simulink model "uvms_sliding"  (Simulink 7.9)
settings: Solver=ode4  StartTime=0.0  StopTime=10.0  FixedStep=dt  RelTol=2*1e-3
values from neighbouring files (symbols this model uses):
  DH = struct('a',zeros(n,1),'d',zeros(n,1),'alpha',zeros(n,1))    [init.m]
  dt = 0.01    [run_simulation.m]
undefined symbols (not defined in the file or in its folder): commanded_zeta, ee_pose_init, Kinetics_Parameters, q_init, V_current, vehicle_euler_init, vehicle_position_init
(part 2 of 2)

== matlab function Controller/sliding mode 2/tau1 ==
  data: Kinetics_Parameters input Bus: kinetics_bus; tau output double; Kinematics input Bus: kin_bus; Measured_States input double; Commanded_States input double; dxi_com input double; dxi_mes input double; dzeta_0_com input double
function tau = slidingMode(Kinetics_Parameters, Kinematics,Measured_States,Commanded_States,dxi_com, dxi_mes, dzeta_0_com)
%#codegen
    Lambda = diag([ones(1,6)*25 , ones(1,6)*25]);
    zeta_mes = Measured_States.zeta;
    y = Lambda * (Commanded_States.xi - Measured_States.xi);
    zeta_0_tilde = dxi_com - dxi_mes;
    zeta_0_com = dxi_com;
    dy = Lambda * zeta_0_tilde;
    s = y + zeta_0_tilde;
    xi_mes = Measured_States.xi;
    
    % get the jacobian Ja
    R0b = Kinematics.Ti.R0b;
    Teuler = getTeuler( Measured_States.xi (4:6)  );
    Ja = [ R0b' , zeros(3,3), zeros(3,6);
           zeros(3,3), Teuler, zeros(3,6);
           zeros(6,3), zeros(6,3), eye(6)
         ];
    dJa = getdJa (Kinematics, zeta_mes, xi_mes, dxi_mes);
    
    N = getN (Kinematics,Kinetics_Parameters);
    M0 = 0.9*getM0 (Kinematics, Kinetics_Parameters, Ja);
    M = getM (Kinematics,Kinetics_Parameters);
    C0 = 1.1*getC0 (Kinematics,Kinetics_Parameters, zeta_mes , Ja, dJa);
    D0 = 1.1*getD0 (Kinematics, Kinetics_Parameters, zeta_mes , Ja);
    
       
    
    Kd=diag([ones(1,6)*60, ones(1,6)*50]);
    Ks=diag([ones(1,6)*390, ones(1,6)*300]);
    
    temp = (dy + dzeta_0_com);
    temp2 = (y + zeta_0_com);
    tau = M0* temp   +  M* dJa* s + C0* temp2 + D0* temp2 + N + Kd*Ja* s + Ks* sat(Ja*s, 0.05);  
    
    
end


function vec = sat (x,epsilon)
    vec=zeros(length(x),1);
    for i=1:length(x)
       if x(i) > epsilon
           vec(i)=1;
       elseif x(i) < -epsilon
           vec(i)=-1;
       else
           vec(i)=x(i)/epsilon;
       end
    end
end

% get the derivative of the jacobian matrix Ja
function dJa = getdJa(Kinematics, zeta, xi , dxi)
    Rb0 = Kinematics.Ti.R0b';
    omega0b = zeta(4:6);
    dRb0 = - Rb0 * skew (omega0b);
    dTb0 = getdTb0( xi, dxi);
    dJa = [ dRb0 , zeros(3,3), zeros(3,6);
           zeros(3,3), dTb0, zeros(3,6);
           zeros(6,3), zeros(6,3), zeros(6,6);
         ];
end

% get the derivative of the Transfromation matrix from euler rates to body
% rates
function dTb0 = getdTb0( xi, dxi)
    dTb0 = zeros(3,3);
    phi = xi(4);
    theta = xi(5);
    dphi = dxi(4);
    dtheta = dxi(5);
    
    dTb0 = [...
            0,           0,      - cos(theta)*dtheta;
            0,    -sin(phi)*dphi,   -sin(theta)*dtheta*sin(phi) + cos(theta)*cos(phi)*dphi;
            0,    -cos(phi)     ,   -sin(theta)*dtheta*cos(phi) - cos(theta)*sin(phi)*dphi
            ];
end

% Get the transformation matrix from euler rates to body rates
function T = getTeuler ( euler )
    phi=euler(1);
    theta=euler(2);
    psi=euler(3);
       
    cphi = cos(phi);
    sphi = sin(phi);
    cth  = cos(theta);
    sth  = sin(theta);
 
    T = [...
      1  0      -sth;
      0  cphi   cth*sphi;
      0  -sphi  cth*cphi ];
end



%% --------------------------------------------------------------
%  Functions to gather the vectors   
%%---------------------------------------------------------------

function M0 = getM0(Kinematics, Kinetics_Parameters, Ja)
    Mrb = getInertiaMatrix(Kinematics, Kinetics_Parameters);
    Ma = getMa(Kinematics, Kinetics_Parameters);
    M0 = (Mrb + Ma)*Ja;
end

function M = getM(Kinematics, Kinetics_Parameters)
    Mrb = getInertiaMatrix(Kinematics, Kinetics_Parameters);
    Ma = getMa(Kinematics, Kinetics_Parameters);
    M = (Mrb + Ma);
end


function C0 = getC0 (Kinematics,Kinetics_Parameters,zeta, Ja, dJa)
    C = getCrb(Kinematics,Kinetics_Parameters, zeta)  + getCa(Kinematics,Kinetics_Parameters,zeta);
    M = getM(Kinematics, Kinetics_Parameters);
    
    C0 = C*Ja + M*dJa;
end

function D0 = getD0 (Kinematics, Kinetics_Parameters,zeta, Ja)
    D =  getD(Kinematics, Kinetics_Parameters,zeta);
    D0 = D* Ja;
end


%% --------------------------------------------------------------
%  Inertia function   
%%---------------------------------------------------------------
function M = getInertiaMatrix(Kinematics, Kinetics_Parameters)
%#codegen
%   getInertiaMatrix Returns the sum of the Rigid body inertia and the added mass:
%   M_rb + M_a
%   
    n=6;
    i=1;
    M = zeros(12,12);
    Inertia = Kinetics_Parameters.Inertia;
    Jgb = [eye(6), zeros(6,6)];                                 % Jacobian from vehicle 
    Ji=Jgb;
    Hi = Kinetics_Parameters.Persistent.Hrg(:,:,i);
    Ii=Hi'*(Inertia(:,:,1))*Hi;                                 % Inertia of vehicle in CO
    M=M+(Ji')*Ii*Ji;
    for i=1:n
        Ji = Kinematics.Ji.Ji(:,:,i);                           % body jacobian
        Hi =Kinetics_Parameters.Persistent.Hrg(:,:,i+1);        % get Transformation matrix of link i
        Ii=Hi'*(Inertia(:,:,i+1) )*Hi;                          % Transform Inertia matrix from CG to CO
        M=M+(Ji')*Ii*Ji;                                        % Add link i's inertia to total inertia
    end
end







%% ------------------------------------------------------
% Persistent Forces   
%%-------------------------------------------------------
function N_p = getN(Kinematics,Kinetics_Parameters)
%#codegen
%   N_p - 12 x 1 vector of generalized forces
%   Persistent_Forces returns the generalized forces due to boyancy and 
%   gravity

    %% init
    n=6;
    N_p=zeros(12,1);
    Jgis = Kinematics.Ji.Ji;
    
    %%  vehicle
    F_bp = getFbp(Kinematics, Kinetics_Parameters,1);           % Get wrench from persistent forces in CO
    Jbb=([eye(6), zeros(6,6)]);                                 % Jacobian from b to b
    N_p = Jbb'*F_bp;                                            % Get contribution to total forces through Jbb
    
    %% robot links
    for i=1:n
        Jgi=Jgis(:,:,i);                                        % Jacobian from b to i
        F_ip = getFip(Kinematics,Kinetics_Parameters, i+1);     % Get wrench in CO
        N_p = N_p + (Jgi')*F_ip;                                % Map to generalized forces and add to total
    end
    N_p = - N_p;                                                % reverse the sign to comply with the sign convention
end
    
    
function F_ip = getFip(Kinematics,Kinetics_Parameters, i)
%#codegen
% function calculating wrench from persistent forces 
% i=b: vehicle
% i>=1: robot arms
    F_ip = zeros(6,1);
    mi = Kinetics_Parameters.Persistent.m(i);
    g = Kinetics_Parameters.Persistent.g;
    rho = Kinetics_Parameters.Persistent.rho;
    nabla = Kinetics_Parameters.Persistent.nabla(i);
    Ri0 = Kinematics.Ti.R0i(:,:,i-1)';
    Hrg = Kinetics_Parameters.Persistent.Hrg(:,:,i);  
    Hrb = Kinetics_Parameters.Persistent.Hrb(:,:,i);
    ez=[0;0;1];
    F_ip(:,:) = (Hrg')*[-mi*g*Ri0*ez ;0;0;0]  + (Hrb')*[rho*nabla*g*Ri0*ez ;0;0;0 ];
end


function F_bp = getFbp(Kinematics,Kinetics_Parameters, i)
%#codegen
% function calculating wrench from persistent forces 
% i=b: vehicle
% i>=1: robot arms
    F_bp = zeros(6,1);
    mi = Kinetics_Parameters.Persistent.m(i);
    g = Kinetics_Parameters.Persistent.g;
    Hrg = Kinetics_Parameters.Persistent.Hrg(:,:,i);  
    Hrb = Kinetics_Parameters.Persistent.Hrb(:,:,i);
    rho = Kinetics_Parameters.Persistent.rho;
    nabla = Kinetics_Parameters.Persistent.nabla(i);
    Ri0 = (Kinematics.Ti.R0b)';
    ez=[0;0;1];
    F_bp(:,:) = (Hrg')*[-mi*g*Ri0*ez ; 0;0;0]  + (Hrb')*[rho*nabla*g*Ri0*ez ; 0;0;0 ];
end

function [phi,theta,psi] = myR2euler(R)
%#codegen
    phi   = atan2(R(3,2),R(3,3));
    theta = -asin(R(3,1));
    psi   = atan2(R(2,1),R(1,1));
end



%% ------------------------------------------------------
% Coriolis Matrix   
%%-------------------------------------------------------
function C = getCrb(Kinematics,Kinetics_Parameters, zeta)
%#codegen
%-----------------------------------------------------------------------
%   This function calculates the coriolis according to From and Pettersen
%   (2013).
%-----------------------------------------------------------------------
    n=6;
    C=zeros(12,12);
    Inertia=Kinetics_Parameters.Inertia;
    Jis = Kinematics.Ji.Ji;
    
    % i = b
    Jgb = [eye(6), zeros(6,6)];
    i=1;
    Hi = Kinetics_Parameters.Persistent.Hrg(:,:,i);
    Ii=Hi'*Inertia(:,:,i);
    Wb = getWb(Ii,zeta);
    C = - (Jgb')*Wb*Hi*Jgb;     % time derivative of Jgb = 0  
    
    % i >=1
    for i=1:n
        Hi = Kinetics_Parameters.Persistent.Hrg(:,:,i+1);
        Ii=Hi'*Inertia(:,:,i+1);
        Wi=getWi(Ii,Jis(:,:,i), zeta);
        Jgi_dot=getJgi_dot(Kinematics, zeta,i);
        Jgi = Jis(:,:,i);
        
        C = C + (Jgi')*Ii*Hi*Jgi_dot - (Jgi')*Wi*Hi*Jgi;
    end
end



function Wb = getWb(I , zeta)
%#codegen
% Get the matrix Wi for i=b
% I: Inertia matrix for vehicle
% zeta: generalized velocity
    Wb = zeros(6,6);
    v = zeta(1:3);
    omega = zeta(4:6);
    mI = I(1:3,1:3); % Identity matrix times mass of link b
    Ib = I(4:6,4:6); % Moment of inertia
    mrgb = I(4:6,1:3); % mass times skew symmetric r_g^b
    dKv= mI*v - mrgb*omega;
    dKomega = Ib*omega + mrgb*v;
    
    Wb = [zeros(3,3), skew(dKv) ; skew(dKv), skew(dKomega)];
end

function Wi = getWi(I, Ji,zeta)
%#codegen
% Get matrix Wi for robot links
% I: inertia matrix for link i
% Ji: Jacobian for link i
% zeta: generalized coordinates
    Wi = zeros(6,6);
    V0i = Ji*zeta;
    v = V0i(1:3);
    omega = V0i(4:6);
    mI = I(1:3,1:3); % Identity matrix times mass of link b
    Ib = I(4:6,4:6); % Moment of inertia
    mrgb = I(4:6,1:3); % mass times skew symmetric r_g^b
    dKv= mI*v - mrgb*omega;
    dKomega = Ib*omega + mrgb*v;
    Wi = [zeros(3,3), skew(dKv) ; skew(dKv), skew(dKomega)];
end

function Jgi_dot=getJgi_dot(Kinematics, zeta,i)
%#codegen
% the functions below is related to Jgi_dot
    Jgi_dot = zeros(6,6+6);
    n=6;
    Jgi = Kinematics.Ji.Ji(:,:,i);
    omega = Jgi*zeta;
    Rbi = Kinematics.Ti.Rbi(:,:,i);
    pbi = Kinematics.Ti.pbi(:,i);
    omegaib = getOmegaib(Kinematics,zeta,i);
    dpbi =  getDpbi(Kinematics,zeta,i);
        
    dAdg_inv = [(Rbi')*skew(omegaib) , -(Rbi')*skew(omegaib)*skew(pbi) + (Rbi')*skew(dpbi); ...
                zeros(3,3) , (Rbi')*skew(omegaib) ];
    dJi = zeros(6,6);
    omega0b = zeta(4:6);
    
    % get d/dt(Ji)
    Xii=[0,0,0,0,0,1]';
    for k=2:n
       if k<=i
            dpbk = getDpbi(Kinematics, zeta ,k-1);
            Rbk= Kinematics.Ti.Rbi(:,:,k-1);
            omega0k = [zeros(3,3) , eye(3)]*Kinematics.Ji.Ji(:,:,k-1)*zeta;
            omegabk = omega0k - (Rbk')*omega0b;
            dJi(:,k) = [zeros(3,3), skew(dpbk)*Rbk*skew(omegabk) ...
                ; zeros(3,3) , (Rbk')*skew(omegabk)]*Xii;
       end
    end
    Ji=getji(Kinematics.Ti, i);
    Adg_inv = Kinematics.Ti.Adgbi_inv(:,:,i);
    Jgi_dot = [dAdg_inv, dAdg_inv*Ji + Adg_inv*dJi ];
end

function omegaib = getOmegaib(Kinematics,zeta,i)
%#codegen
% returns angular rage of vehcile wrt frame i noted in vehicle frame
    omegaib = zeros(3,1);
    Rbi = Kinematics.Ti.Rbi(:,:,i);
    Jgi = Kinematics.Ji.Ji(:,:,i);
    omega0b = zeta(4:6);
    omegaib = omega0b - Rbi*[zeros(3,3), eye(3)]*Jgi*zeta;
end

function dpbi = getDpbi( Kinematics, zeta,iter)
%#codegen
% returns time derivative of position vector of from frame b to frame i
    dpbi = zeros(3,1);
    H = [eye(3), zeros(3,3)];
    Rbi=Kinematics.Ti.Rbi(:,:,iter);
    Adgbi_inv = Kinematics.Ti.Adgbi_inv(:,:,iter);
    Ji = getji(Kinematics.Ti,iter);
    qd=zeros(6,1);
    qd(:,:)=zeta(7:12);
    dpbi = Rbi*H*Adgbi_inv*Ji*qd;
end


function mat = getji(Ti,i)
%#codegen
% return matrix Ji (see report)
    n=6;
    mat=zeros(6,6);
    Xii=[0,0,0,0,0,1]';
    mat(:,1)=eye(6)*Xii;
    for j=2:n
        if j<=i
            mat(:,j) = Ti.Adgbi(:,:,j-1)*Xii;
        end
    end
end

function S = skew(v)
%#codegen

  S = [  0   -v(3)  v(2)
       v(3)  0    -v(1)
       -v(2) v(1)   0];
end


%% ------------------------------------------------------
% D matrix 
%%-------------------------------------------------------
function D = getD(Kinematics, Kinetics_Parameters,zeta_r)
%#codegen
%
% Returns the D matrix in the dynamics equation. The total forces is based
% on mappin the forces in each frame to the total generalized forces
% through the jacoian: tau = J^T*F_i. The forces in frame i is calculated
% from the forces in CG to CO through the transformation matrix: F_co =
% Hrg^T*F_cg
%
    %% init
    n=6;
    D=zeros(12,12);                                      % init matrix size
    HydroDynamics = Kinetics_Parameters.HydroDynamics;   % Hydrodynamics parameters
    Jgis = Kinematics.Ji.Ji;                             % Jacobians
    Hrgs = Kinetics_Parameters.Persistent.Hrg;           % Transformation matrix
    
    
    %% vehicle
    i=1;
    Jbb=[eye(6), zeros(6)];                               % Jacobian from frame 0 to frame b
    Hrg = Hrgs(:,:,i);                                    % Transformation matrix
    Vcg = Hrg*Jbb*zeta_r;                                   % velocity in CG mapped from CO
    Dcg =  HydroDynamics.Linear(:,:,i) + ...
           HydroDynamics.Quadratic(:,:,i)*diag(abs(Vcg)); % Wrench in CG
    Di = Hrg'*Dcg;                                        % Wrench in CO mapped from CG    
    D = Jbb'*Di*Jbb;                                      % Add contribution to the total matrix mapped from frame i 
                                                          % to generalized coordinates                                   
    
    %% robot links
    for i=1:n
        Jgi = Jgis(:,:,i);                                % Jacobian from frame 0 to frame i 
        Hrg = Hrgs(:,:,i+1);                              % Transformation matrix
        Vcg = Hrg*Jgi*zeta_r;                               % velocity in CG
        Dcg = HydroDynamics.Linear(:,:,i+1)+... 
          HydroDynamics.Quadratic(:,:,i+1)*diag(abs(Vcg));% Wrench in CG   
        Di = Hrg'*Dcg;                                    % Wrench in CO    
        D = D + Jgi'*Di*Jgi;                              % Add frame i's contribution to D matrix    
    end
end

%% ------------------------------------------------------
% Added Coriolis
%%-------------------------------------------------------
function Ca = getCa(Kinematics,Kinetics_Parameters,zeta_r)
%%#codegen ..............................................
%
%   This function calculates the added coriolis matrix
%.......................................................
    n=6;
    Ca=zeros(12,12);
    Inertia=Kinetics_Parameters.AddedInertia;
    Jis = Kinematics.Ji.Ji;
    
    % vehicle
    Jgb = [eye(6), zeros(6,6)];
    i=1;
    Hi = Kinetics_Parameters.Persistent.Hrg(:,:,i+1);
    Ii=Hi'*Inertia(:,:,i);
    Wb = getWb(Ii,zeta_r);
    Ca = - (Jgb')*Wb*Hi*Jgb;     % time derivative of Jgb = 0  
    
    % manipulator links
    for i=1:n
        Hi = Kinetics_Parameters.Persistent.Hrg(:,:,i+1);
        Ii=Hi'*Inertia(:,:,i+1);
        Wi=getWi(Ii,Jis(:,:,i), zeta_r);
        Jgi_dot=getJgi_dot(Kinematics, zeta_r,i);
        Jgi = Jis(:,:,i);
        Ca = Ca + (Jgi')*Ii*Hi*Jgi_dot - (Jgi')*Wi*Hi*Jgi;
    end
end

%% ------------------------------------------------------
% Added Mass
%%-------------------------------------------------------
function Ma = getMa(Kinematics,Kinetics_Parameters)
%#codegen ..........................
%
%  returns rest of the the added mass
%  force matrix:
%       Ma*H(xi,zeta)
% ..................................
    n=6;
    i=1;
    
    %% get the total Added mass matrix
    Ma = zeros(12,12);
    AddedInertia = Kinetics_Parameters.AddedInertia;
    Jgb = [eye(6), zeros(6,6)];                                 % Jacobian from vehicle 
    Ji=Jgb;
    Hi = Kinetics_Parameters.Persistent.Hrg(:,:,i);
    Ii=Hi'*( AddedInertia(:,:,1))*Hi;                           % Inertia of vehicle in CO
    Ma=Ma+(Ji')*Ii*Ji;
    for i=1:n
        Ji = Kinematics.Ji.Ji(:,:,i);                           % body jacobian
        Hi =Kinetics_Parameters.Persistent.Hrg(:,:,i+1);        % get Transformation matrix of link i
        Ii=Hi'*(AddedInertia(:,:,i+1))*Hi;                      % Transform Inertia matrix from CG to CO
        Ma=Ma+(Ji')*Ii*Ji;                                      % Add link i's inertia to total inertia
    end
 end
